simulink model "ExtremumSeekingControlExample"  (R2021a)
settings: Solver=FixedStepAuto  StartTime=0.0  StopTime=T  FixedStep=Ts  RelTol=1e-3
values from neighbouring files (symbols this model uses):
  D_A = 1    [ExtremumSeekingControlExample_m.m]
  D_w = 0.4    [ExtremumSeekingControlExample_m.m]
  M_A = 2/D_A    (= 2)    [ExtremumSeekingControlExample_m.m]
  M_phi = 0/180*pi    (= 0)    [ExtremumSeekingControlExample_m.m]
  M_w = D_w    (= 0.4)    [ExtremumSeekingControlExample_m.m]
  Ts = 0.1    [ExtremumSeekingControlExample_m.m]
  w_A = 0.5    [ExtremumSeekingControlExample_m.m]
  x_off = 5    [ExtremumSeekingControlExample_m.m]
  y_off = -10    [ExtremumSeekingControlExample_m.m]
undefined symbols (not defined in the file or in its folder): DiscIntNeverNeededParam
libraries: DRC_SimulinkLibrary x2
settings Model: Creator=sebastiaanmuld  LastModifiedBy=sebastiaanmuld

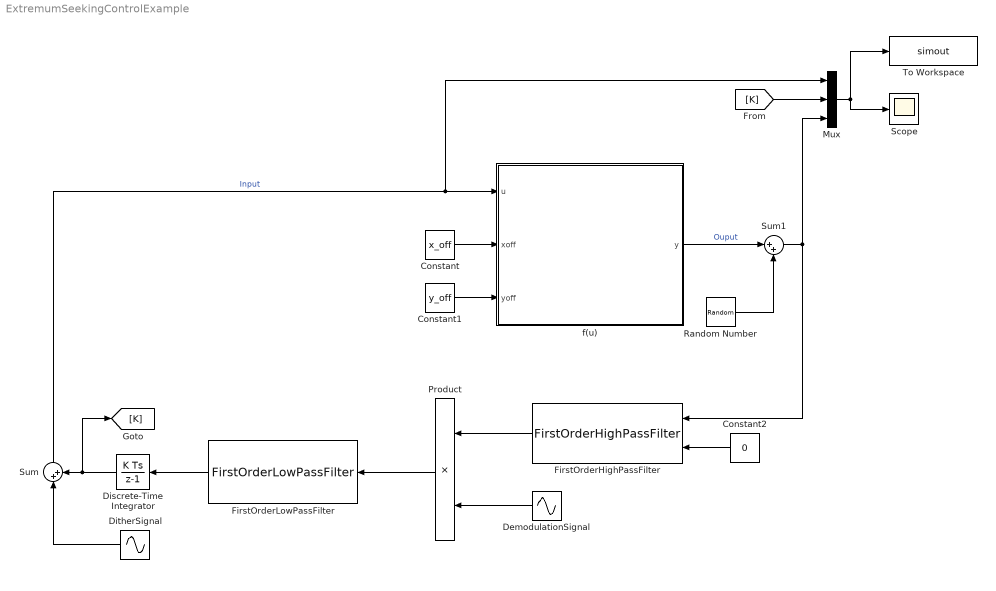
== system ExtremumSeekingControlExample ==
  Constant : Constant  Value=x_off
  Constant1 : Constant  Value=y_off
  Constant2 : Constant  Value=0
  DemodulationSignal : Sin  Amplitude=M_A  Frequency=M_w  Phase=M_phi  SampleTime=Ts
  Discrete-Time Integrator : DiscreteIntegrator  gainval=Ki  SampleTime=-1  ICPrevOutput=DiscIntNeverNeededParam  ICPrevScaledInput=DiscIntNeverNeededParam
  DitherSignal : Sin  Amplitude=D_A  Frequency=D_w  SampleTime=Ts
  FirstOrderHighPassFilter : DRC_SimulinkLibrary/FirstOrderHighPassFilter  wc=F.wcHPF  Ts=Ts
  FirstOrderLowPassFilter : DRC_SimulinkLibrary/FirstOrderLowPassFilter  wn=F.wcLPF  Ts=Ts
  Mux : Mux  Inputs=3
  Product : Product
  Random Number : RandomNumber  Variance=w_A  SampleTime=Ts
  Scope : Scope
  Sum : Sum  Inputs=|++
  Sum1 : Sum  Inputs=|++
  To Workspace : ToWorkspace  VariableName=simout  SaveFormat=Timeseries  SampleTime=-1
  f(u) : MATLAB Function  TreatAsAtomicUnit=on
  wires:
  Constant/1 -> f(u)/2(xoff)
  Constant1/1 -> f(u)/3(yoff)
  Constant2/1 -> FirstOrderHighPassFilter/2
  FirstOrderHighPassFilter/1 -> Product/1
  DemodulationSignal/1 -> Product/2
  Product/1 -> FirstOrderLowPassFilter/1
  FirstOrderLowPassFilter/1 -> Discrete-Time Integrator/1
  Discrete-Time Integrator/1 -> [K], Sum/2
  DitherSignal/1 -> Sum/1
  Sum/1 -> Mux/1, f(u)/1(u)  "Input"
  Mux/1 -> Scope/1, To Workspace/1
  Random Number/1 -> Sum1/2
  f(u)/1(y) -> Sum1/1  "Ouput"
  Sum1/1 -> FirstOrderHighPassFilter/1, Mux/3
  [K] -> Mux/2

== matlab function ExtremumSeekingControlExample/f(u) ==
  data: u input; y output; xoff input; yoff input
function y = P(u, xoff, yoff)

    y = -(u-xoff)^2 + yoff;
    
end
